simulink model "pd_control"  (R2015b)
settings: Solver=VariableStepAuto  StartTime=0.0  StopTime=stop_time  RelTol=1e-6
values from neighbouring files (symbols this model uses):
  theta_0 = 0    [main_nonlinear_spacecraft_euler.m]    (also in main_on_off_thruster.m = 2; main_reaction_wheels_design_v03.m = -0.3; main_reaction_wheels_design_v04.m = -0.10471975512)
undefined symbols (not defined in the file or in its folder): I, k_d, k_p, omega_0
settings Model: Creator=Krunal's PC  LastModifiedBy=Krunal's PC

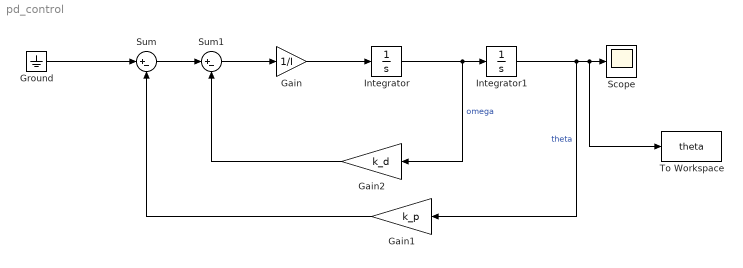
== system pd_control ==
  Gain : Gain  Gain=1/I
  Gain1 : Gain  Gain=k_p
  Gain2 : Gain  Gain=k_d
  Ground : Ground
  Integrator : Integrator  InitialCondition=omega_0
  Integrator1 : Integrator  InitialCondition=theta_0
  Scope : Scope
  Sum : Sum  Inputs=|+-
  Sum1 : Sum  Inputs=|+-
  To Workspace : ToWorkspace  VariableName=theta  SampleTime=-1
  wires:
  Sum/1 -> Sum1/1
  Sum1/1 -> Gain/1
  Gain/1 -> Integrator/1
  Integrator/1 -> Gain2/1, Integrator1/1  "omega"
  Integrator1/1 -> Gain1/1, To Workspace/1, Scope/1  "theta"
  Gain1/1 -> Sum/2
  Gain2/1 -> Sum1/2
  Ground/1 -> Sum/1
